simulink model "flatball_6dof"  (R2021b)
settings: Solver=ode1be  StartTime=0.0  StopTime=30  FixedStep=1e-3  MaxStep=0.01  MinStep=0.01  RelTol=1e-3
values from neighbouring files (symbols this model uses):
  amb = evalin( 'base', 'amb')    [flatball_6dof_eqom.m]
  C = evalin( 'base', 'C')    [flatball_6dof_eqom.m]
  disc = evalin( 'base', 'disc')    [flatball_6dof_eqom.m]    (also in flatball_6dof_init.m = struct; flatball_init_disc_params.m = struct)
  X0_z1m_at_rest = [1e-3 1e-3 -1, -1e-6 1e-6 -1e-6, 0 0 1e-6, 0 0 -1e-6]    [flatball_6dof_wrk.m]    (also in hummel_thesis_mdl_validation.m)
undefined symbols (not defined in the file or in its folder): clock, flatball, flatball_6dof_plnt_lib, HandH
libraries: simulink x6, aerolibanim x3, aerolibnav x3, matrix_library x3, mspfiltlib x1, hucker_lib x1
(part 2 of 3)

== system flatball_6dof/flatball-6dof-HandH/calc-F-M/lab/calc-M/q-inf ==
  X : Inport
  Gain : Gain  Gain=0.5
  Product1 : Product  Inputs=3
  Product2 : Product
  S : Constant  Value=disc.A
  Square : Math  Operator=square  SaturateOnIntegerOverflow=on
  X-to-vel : MATLAB Function  TreatAsAtomicUnit=on
  d : Constant  Value=disc.d
  rho : Constant  Value=amb.rho
  vector-norm : MATLAB Function  TreatAsAtomicUnit=on
  q-inf-S : Outport
  q-inf-S-d : Outport  Port=2
  wires:
  d/1 -> Product2/2
  Product2/1 -> q-inf-S-d/1
  X-to-vel/1(vel) -> vector-norm/1(vec)
  Gain/1 -> q-inf-S/1, Product2/1
  Square/1 -> Product1/1
  S/1 -> Product1/2
  vector-norm/1(norm) -> Square/1
  X/1 -> X-to-vel/1(X)
  rho/1 -> Product1/3
  Product1/1 -> Gain/1

== system flatball_6dof/flatball-6dof-HandH/calc-F-M/lab/helpers/Subsystem ==
  Xdot : Inport
  Display : Display
  Gain : Gain  Gain=-1
  Ground2 : Ground
  Ground3 : Ground
  Ta1 : MATLAB Function  TreatAsAtomicUnit=on
  zero-side-slip-angle : MATLAB Function  TreatAsAtomicUnit=on
  Ta23 : Outport
  wires:
  Ground2/1 -> Ta1/2(theta)
  Gain/1 -> Ta1/3(psi)
  Ground3/1 -> Ta1/1(phi)
  Ta1/1(T) -> Ta23/1  "Ta23"
  zero-side-slip-angle/1(beta) -> Display/1, Gain/1  "beta"
  Xdot/1 -> zero-side-slip-angle/1(Xdot)

== system flatball_6dof/flatball-6dof-HandH/calc-F-M/lab/helpers/Subsystem1 ==
  X1_dot : Inport
  TH1_dot : Inport  Port=2
  TH1 : Inport  Port=3
  Display : Display
  Display1 : Display
  MatrixMultiply : Product  Multiplication=Matrix(*)
  MatrixMultiply1 : Product  Multiplication=Matrix(*)
  transformation-matrices : Subsystem
  w_ : MATLAB Function  TreatAsAtomicUnit=on
  X2_dot : Outport
  TH2_dot : Outport  Port=2
  w~ : Outport  Port=3
  wires:
  MatrixMultiply/1 -> Display/1, X2_dot/1
  MatrixMultiply1/1 -> w_/1(THdot), Display1/1, TH2_dot/1
  transformation-matrices/1(Ta12) -> MatrixMultiply/1
  transformation-matrices/2(Tr12) -> MatrixMultiply1/1
  X1_dot/1 -> MatrixMultiply/2
  TH1_dot/1 -> MatrixMultiply1/2
  TH1/1 -> transformation-matrices/1(TH)
  w_/1(M) -> w~/1  "w_"

== system flatball_6dof/flatball-6dof-HandH/calc-F-M/lab/helpers/Subsystem2 ==
  Xdot : Inport
  Display : Display
  Ground : Ground
  Ground1 : Ground
  Ta2 : MATLAB Function  TreatAsAtomicUnit=on
  angle-of-attack : MATLAB Function  TreatAsAtomicUnit=on
  Ta34 : Outport
  wires:
  Ground1/1 -> Ta2/3(psi)
  Ta2/1(T) -> Ta34/1  "Ta34"
  angle-of-attack/1(alpha) -> Display/1, Ta2/2(theta)  "alpha"
  Xdot/1 -> angle-of-attack/1(Xdot)
  Ground/1 -> Ta2/1(phi)

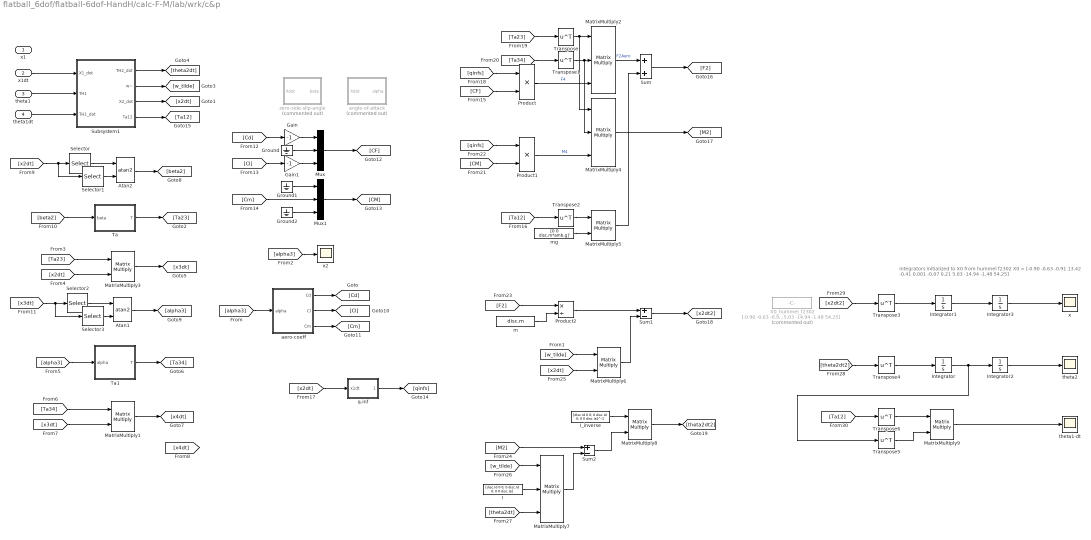
== system flatball_6dof/flatball-6dof-HandH/calc-F-M/lab/wrk/c&p ==
  note: integrators initialized to X0 from hummel f2302
      | X0 = [-0.90 -0.63 -0.91 13.42 -0.41 0.001 -0.07 0.21 5.03 -14.94 -1.48 54.25]
  x1 : Inport
  x1dt : Inport  Port=2
  theta1 : Inport  Port=3
  theta1dt : Inport  Port=4
  Atan1 : Trigonometry  Operator=atan2
  Atan2 : Trigonometry  Operator=atan2
  Gain : Gain  Gain=-1
  Gain1 : Gain  Gain=-1
  Ground : Ground
  Ground1 : Ground
  Ground2 : Ground
  I : Constant  Value=[disc.Id 0 0; 0 disc.Id 0; 0 0 disc.Ia]
  I_inverse : Constant  Value=[disc.Id 0 0; 0 disc.Id 0; 0 0 disc.Ia]^-1
  Integrator : Integrator  InitialCondition=[-14.94 -1.48 54.25]
  Integrator1 : Integrator  InitialCondition=[13.42 -0.41 0.001]
  Integrator2 : Integrator  InitialCondition=[-0.07 0.21 5.03]
  Integrator3 : Integrator  InitialCondition=[-0.90 -0.63 -0.91]
  MatrixMultiply{1,3,5..6,8..9} (6 alike) : Product  Multiplication=Matrix(*)
  MatrixMultiply2 : Product  Inputs=3  Multiplication=Matrix(*)
  MatrixMultiply4 : Product  Inputs=3  Multiplication=Matrix(*)
  MatrixMultiply7 : Product  Inputs=3  Multiplication=Matrix(*)
  Mux : Mux  Inputs=3
  Mux1 : Mux  Inputs=3
  Product : Product
  Product1 : Product
  Product2 : Product  Inputs=*/
  Selector : Selector  InputPortWidth=3  IndexOptions=Index vector (dialog)  Indices=[2]  OutputSizes=1
  Selector1 : Selector  InputPortWidth=3  IndexOptions=Index vector (dialog)  Indices=[1]  OutputSizes=1
  Selector2 : Selector  InputPortWidth=3  IndexOptions=Index vector (dialog)  Indices=[3]  OutputSizes=1
  Selector3 : Selector  InputPortWidth=3  IndexOptions=Index vector (dialog)  Indices=[1]  OutputSizes=1
  Subsystem1 : Subsystem
  Sum : Sum
  Sum1 : Sum  Inputs=+-
  Sum2 : Sum  Inputs=+-
  Ta : MATLAB Function  TreatAsAtomicUnit=on
  Ta1 : MATLAB Function  TreatAsAtomicUnit=on
  Transpose{,1..6} (7 alike) : Math  Operator=transpose  SaturateOnIntegerOverflow=on
  X0_hummel_f2302 : Constant  Commented=on  Value=[-0.90 -0.63 -0.91 13.42 -0.41 0.001 -0.07 0.21 5.03 -14.94 -1.48 54.25]
  aero-coeff : Subsystem
  angle-of-attack : MATLAB Function  Commented=on  TreatAsAtomicUnit=on
  m : Constant  Value=disc.m
  mg : Constant  Value=[0 0 disc.m*amb.g]'
  q-inf : Subsystem
  theta1-dt : Scope
  theta2 : Scope
  x : Scope
  x2 : Scope
  zero-side-slip-angle : MATLAB Function  Commented=on  TreatAsAtomicUnit=on
  wires:
  x1dt/1 -> Subsystem1/1(X1_dot)
  theta1dt/1 -> Subsystem1/3(TH1_dot)
  theta1/1 -> Subsystem1/2(TH1)
  Ta/1(T) -> [Ta23]
  Subsystem1/2(w~) -> [w_tilde]
  Subsystem1/1(TH2_dot) -> [theta2dt]
  [beta2] -> Ta/1(beta)
  MatrixMultiply3/1 -> [x3dt]
  [alpha3] -> Ta1/1(alpha)
  Ta1/1(T) -> [Ta34]
  MatrixMultiply1/1 -> [x4dt]
  [x2dt] -> Selector1/1, Selector/1
  Atan2/1 -> [beta2]
  Atan1/1 -> [alpha3]
  aero-coeff/1(Cd) -> [Cd]
  aero-coeff/3(Cm) -> [Cm]
  aero-coeff/2(Cl) -> [Cl]
  [alpha3] -> aero-coeff/1(alpha)
  [Cd] -> Gain/1
  [Cl] -> Gain1/1
  Ground/1 -> Mux/2
  Mux/1 -> [CF]
  Gain/1 -> Mux/1
  Gain1/1 -> Mux/3
  [Cm] -> Mux1/2
  Ground1/1 -> Mux1/1
  Ground2/1 -> Mux1/3
  Mux1/1 -> [CM]
  [x2dt] -> q-inf/1(x1dt)
  q-inf/1(q-inf-S) -> [qinfs]
  [qinfs] -> Product/1
  [CF] -> Product/2
  [Ta34] -> Transpose1/1
  [Ta23] -> Transpose/1
  Transpose/1 -> MatrixMultiply4/1, MatrixMultiply2/1
  Transpose1/1 -> MatrixMultiply4/2, MatrixMultiply2/2
  Product/1 -> MatrixMultiply2/3  "F4"
  [CM] -> Product1/2
  [qinfs] -> Product1/1
  Product1/1 -> MatrixMultiply4/3  "M4"
  [Ta23] -> MatrixMultiply3/1
  [x2dt] -> MatrixMultiply3/2
  [x3dt] -> MatrixMultiply1/2
  [Ta34] -> MatrixMultiply1/1
  Subsystem1/4(Ta12) -> [Ta12]
  [Ta12] -> Transpose2/1
  Transpose2/1 -> MatrixMultiply5/1
  mg/1 -> MatrixMultiply5/2
  MatrixMultiply2/1 -> Sum/1  "F2Aero"
  MatrixMultiply5/1 -> Sum/2
  Sum/1 -> [F2]
  MatrixMultiply4/1 -> [M2]
  [F2] -> Product2/1
  m/1 -> Product2/2
  Product2/1 -> Sum1/1
  [w_tilde] -> MatrixMultiply6/1
  [x2dt] -> MatrixMultiply6/2
  MatrixMultiply6/1 -> Sum1/2
  Sum1/1 -> [x2dt2]
  [M2] -> Sum2/1
  [theta2dt] -> MatrixMultiply7/3
  [w_tilde] -> MatrixMultiply7/1
  I/1 -> MatrixMultiply7/2
  MatrixMultiply7/1 -> Sum2/2
  MatrixMultiply8/1 -> [theta2dt2]
  [theta2dt2] -> Transpose4/1
  [x2dt2] -> Transpose3/1
  Integrator/1 -> Integrator2/1, Transpose5/1
  Integrator1/1 -> Integrator3/1
  Integrator2/1 -> theta2/1
  Integrator3/1 -> x/1
  I_inverse/1 -> MatrixMultiply8/1
  Sum2/1 -> MatrixMultiply8/2
  Subsystem1/3(X2_dot) -> [x2dt]
  Transpose3/1 -> Integrator1/1
  Transpose4/1 -> Integrator/1
  [alpha3] -> x2/1
  Selector/1 -> Atan2/1
  Selector1/1 -> Atan2/2
  Selector3/1 -> Atan1/2
  Selector2/1 -> Atan1/1
  [x3dt] -> Selector3/1, Selector2/1
  Transpose5/1 -> MatrixMultiply9/2
  [Ta12] -> Transpose6/1
  Transpose6/1 -> MatrixMultiply9/1
  MatrixMultiply9/1 -> theta1-dt/1

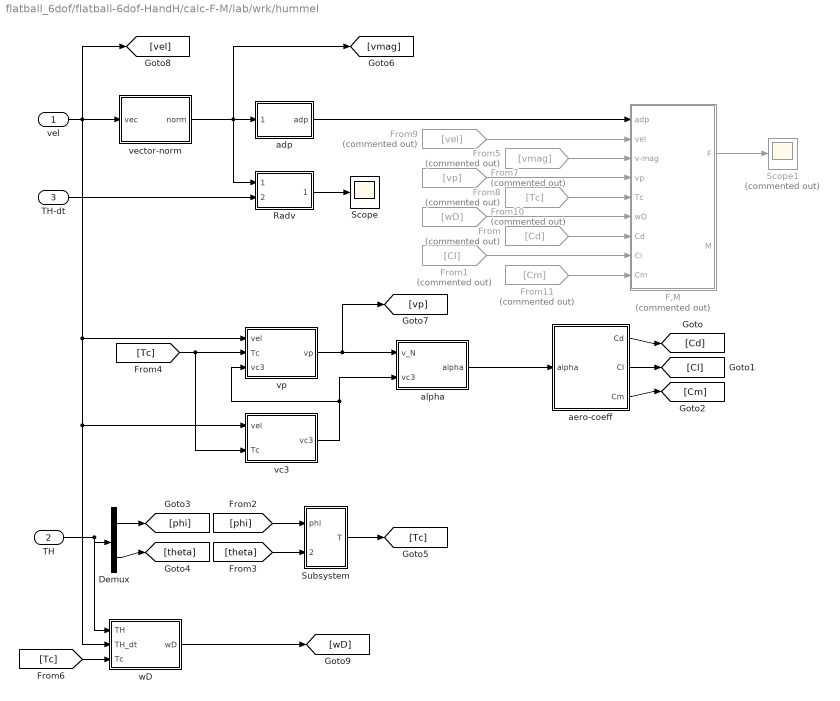
== system flatball_6dof/flatball-6dof-HandH/calc-F-M/lab/wrk/hummel ==
  vel : Inport
  TH : Inport  Port=2
  TH-dt : Inport  Port=3
  Demux : Demux  Outputs=2
  F,M : Subsystem  Commented=on
  From : From  Commented=on  GotoTag=Cd
  From1 : From  Commented=on  GotoTag=Cl
  From10 : From  Commented=on  GotoTag=wD
  From11 : From  Commented=on  GotoTag=Cm
  From5 : From  Commented=on  GotoTag=vmag
  From7 : From  Commented=on  GotoTag=vp
  From8 : From  Commented=on  GotoTag=Tc
  From9 : From  Commented=on  GotoTag=vel
  Radv : Subsystem
  Scope : Scope
  Scope1 : Scope  Commented=on
  Subsystem : Subsystem
  adp : Subsystem
  aero-coeff : Subsystem
  alpha : MATLAB Function  TreatAsAtomicUnit=on
  vc3 : MATLAB Function  TreatAsAtomicUnit=on
  vector-norm : MATLAB Function  TreatAsAtomicUnit=on
  vp : MATLAB Function  TreatAsAtomicUnit=on
  wD : MATLAB Function  TreatAsAtomicUnit=on
  wires:
  aero-coeff/1(Cd) -> [Cd]
  aero-coeff/2(Cl) -> [Cl]
  aero-coeff/3(Cm) -> [Cm]
  adp/1(adp) -> F,M/1(adp)
  vel/1 -> [vel], wD/2(TH_dt), vc3/1(vel), vp/1(vel), vector-norm/1(vec)
  TH/1 -> wD/1(TH), Demux/1
  Demux/2 -> [theta]
  Demux/1 -> [phi]
  [phi] -> Subsystem/1(phi)
  [theta] -> Subsystem/2(theta)
  vector-norm/1(norm) -> Radv/1(v-mag), [vmag], adp/1(v-mag)
  Subsystem/1(T) -> [Tc]
  vp/1(vp) -> [vp], alpha/1(v_N)
  [Tc] -> vc3/2(Tc), vp/2(Tc)
  vc3/1(vc3) -> vp/3(vc3), alpha/2(vc3)
  alpha/1(alpha) -> aero-coeff/1(alpha)
  TH-dt/1 -> Radv/2(TH-dt)
  Radv/1(Radv) -> Scope/1
  [Tc] -> wD/3(Tc)
  wD/1(wD) -> [wD]
  From5/1 -> F,M/3(v-mag)
  From7/1 -> F,M/4(vp)
  From8/1 -> F,M/5(Tc)
  F,M/1(F) -> Scope1/1
  From9/1 -> F,M/2(vel)
  From10/1 -> F,M/6(wD)
  From/1 -> F,M/7(Cd)
  From1/1 -> F,M/8(Cl)
  From11/1 -> F,M/9(Cm)

== system flatball_6dof/flatball-6dof-HandH/scopes/work-in-progress/body-forces-and-moments/mg ==
  Constant1 : Constant  Value=amb.g
  Constant2 : Constant  Value=disc.m
  Ground4 : Ground
  Ground5 : Ground
  Mux2 : Mux  Inputs=3
  Product4 : Product
  mg : Outport
  wires:
  Product4/1 -> mg/1
  Constant1/1 -> Mux2/3
  Ground4/1 -> Mux2/1
  Constant2/1 -> Product4/1
  Mux2/1 -> Product4/2
  Ground5/1 -> Mux2/2

== system flatball_6dof/flatball-6dof-HandH/scopes/work-in-progress/earth-reference/beta2 ==
  X2dot : Inport
  Atan2 : Trigonometry  Operator=atan2
  Selector : Selector  InputPortWidth=3  IndexOptions=Index vector (dialog)  Indices=[2]  OutputSizes=1
  Selector3 : Selector  InputPortWidth=3  IndexOptions=Index vector (dialog)  Indices=[1]  OutputSizes=1
  tag scope: beta2=scoped
  wires:
  Atan2/1 -> [beta2]
  Selector/1 -> Atan2/1  "v2"
  Selector3/1 -> Atan2/2  "u2"
  X2dot/1 -> Selector3/1, Selector/1

== system flatball_6dof/flatball-6dof-HandH/scopes/work-in-progress/earth-reference/v_inf ==
  X2dot : Inport
  Demux : Demux  Outputs=3
  Sqrt : Sqrt  SaturateOnIntegerOverflow=on
  Square : Math  Operator=square  SaturateOnIntegerOverflow=on
  Square1 : Math  Operator=square  SaturateOnIntegerOverflow=on
  Square2 : Math  Operator=square  SaturateOnIntegerOverflow=on
  Sum : Sum  Inputs=3
  tag scope: v_inf=scoped
  wires:
  Square1/1 -> Sum/2
  Square2/1 -> Sum/3
  Sum/1 -> Sqrt/1
  Demux/1 -> Square/1
  Square/1 -> Sum/1
  Demux/3 -> Square2/1
  X2dot/1 -> Demux/1
  Demux/2 -> Square1/1
  Sqrt/1 -> [v_inf]

== system flatball_6dof/flatball-6dof-HandH/scopes/work-in-progress/earth-reference/w_tilde ==
  X2dot : Inport
  MATLAB Function : MATLAB Function  TreatAsAtomicUnit=on
  tag scope: w_tilde=scoped
  wires:
  MATLAB Function/1(w) -> [w_tilde]
  X2dot/1 -> MATLAB Function/1(X2dot)

== system flatball_6dof/flatball-6dof-HandH/scopes/work-in-progress/eml-6dof/lab ==
  X1 : Inport
  TH1 : Inport  Port=2
  X1-dot : Inport  Port=3
  TH1-dot : Inport  Port=4
  X2-dot : Inport  Port=5
  TH2-dot : Inport  Port=6
  X3-dot : Inport  Port=7
  TH3-dot : Inport  Port=8
  alpha3 : Inport  Port=9
  beta2 : Inport  Port=10
  Compare To Constant : simulink/Logic and Bit Operations/Compare To Constant  relop=>=  const=0.0  OutDataTypeStr=boolean
  Gain : Gain  Gain=C.RAD2DEG
  Gain1 : Gain  Gain=C.RAD2DEG
  Scope{,1..9} (10 alike) : Scope
  Selector : Selector  InputPortWidth=3  IndexOptions=Index vector (dialog)  Indices=[3]  OutputSizes=1
  Selector1 : Selector  InputPortWidth=3  IndexOptions=Index vector (dialog)  Indices=[1 2]  OutputSizes=1
  Stop Simulation : Stop
  wires:
  Selector1/1 -> Scope1/1
  Gain1/1 -> Scope9/1
  Gain/1 -> Scope8/1
  Selector/1 -> Compare To Constant/1
  Compare To Constant/1 -> Stop Simulation/1
  TH3-dot/1 -> Scope7/1
  TH1-dot/1 -> Scope3/1
  TH2-dot/1 -> Scope5/1
  X2-dot/1 -> Scope4/1
  TH1/1 -> Selector1/1
  X1/1 -> Scope/1, Selector/1
  beta2/1 -> Gain1/1
  X3-dot/1 -> Scope6/1
  X1-dot/1 -> Scope2/1
  alpha3/1 -> Gain/1

== system flatball_6dof/flatball-6dof-HandH/calc-F-M/lab/calc-F/aero-coeff/Subsystem ==
  alpha : Inport
  Cd0 : Constant  Value=disc.CD0
  Cda : Constant  Value=disc.CDa
  Product : Product
  Square : Math  Operator=square  SaturateOnIntegerOverflow=on
  Sum : Sum
  Sum1 : Sum
  alpha0 : Constant  Value=disc.alpha0
  Cd : Outport
  wires:
  Sum1/1 -> Cd/1
  Square/1 -> Product/2
  Product/1 -> Sum1/2
  Cda/1 -> Product/1
  Cd0/1 -> Sum1/1
  Sum/1 -> Square/1
  alpha0/1 -> Sum/2
  alpha/1 -> Sum/1

== system flatball_6dof/flatball-6dof-HandH/calc-F-M/lab/calc-F/aero-coeff/Subsystem1 ==
  alpha : Inport
  CL0 : Constant  Value=disc.CL0
  CLa : Constant  Value=disc.CLa
  Product : Product
  Sum1 : Sum
  Cl : Outport
  wires:
  alpha/1 -> Product/2
  CL0/1 -> Sum1/1
  CLa/1 -> Product/1
  Product/1 -> Sum1/2
  Sum1/1 -> Cl/1

== system flatball_6dof/flatball-6dof-HandH/calc-F-M/lab/calc-M/aero-coeff/Subsystem2 ==
  alpha : Inport
  CM0 : Constant  Value=disc.CM0
  CMa : Constant  Value=disc.CMa
  Product : Product
  Sum1 : Sum
  Cm : Outport
  wires:
  Sum1/1 -> Cm/1
  Product/1 -> Sum1/2
  CMa/1 -> Product/1
  CM0/1 -> Sum1/1
  alpha/1 -> Product/2

== system flatball_6dof/flatball-6dof-HandH/calc-F-M/lab/helpers/Subsystem1/transformation-matrices ==
  TH : Inport
  Ta : MATLAB Function  TreatAsAtomicUnit=on
  Tr : MATLAB Function  TreatAsAtomicUnit=on
  Ta12 : Outport
  Tr12 : Outport  Port=2
  wires:
  TH/1 -> Ta/1(TH), Tr/1(TH)
  Ta/1(M) -> Ta12/1  "Ta12"
  Tr/1(M) -> Tr12/1  "Tr12"

== system flatball_6dof/flatball-6dof-HandH/calc-F-M/lab/wrk/c&p/Subsystem1 ==
  X1_dot : Inport
  TH1 : Inport  Port=2
  TH1_dot : Inport  Port=3
  MatrixMultiply : Product  Multiplication=Matrix(*)
  MatrixMultiply1 : Product  Multiplication=Matrix(*)
  Transpose : Math  Operator=transpose  SaturateOnIntegerOverflow=on
  Transpose1 : Math  Operator=transpose  SaturateOnIntegerOverflow=on
  transformation-matrices : Subsystem
  w_ : MATLAB Function  TreatAsAtomicUnit=on
  TH2_dot : Outport
  w~ : Outport  Port=2
  X2_dot : Outport  Port=3
  Ta12 : Outport  Port=4
  wires:
  MatrixMultiply/1 -> X2_dot/1
  MatrixMultiply1/1 -> w_/1(THdot), TH2_dot/1
  transformation-matrices/1(Ta12) -> Transpose/1, Ta12/1
  transformation-matrices/2(Tr12) -> Transpose1/1
  X1_dot/1 -> MatrixMultiply/2
  TH1_dot/1 -> MatrixMultiply1/2
  TH1/1 -> transformation-matrices/1(TH)
  w_/1(M) -> w~/1  "w_"
  Transpose/1 -> MatrixMultiply/1  "Ta21"
  Transpose1/1 -> MatrixMultiply1/1  "Ta21"

== system flatball_6dof/flatball-6dof-HandH/calc-F-M/lab/wrk/c&p/aero-coeff ==
  alpha : Inport
  Subsystem : Subsystem
  Subsystem1 : Subsystem
  Subsystem2 : Subsystem
  Cd : Outport
  Cl : Outport  Port=2
  Cm : Outport  Port=3
  wires:
  alpha/1 -> Subsystem2/1(alpha), Subsystem1/1(alpha), Subsystem/1(alpha)
  Subsystem2/1(Cm) -> Cm/1
  Subsystem1/1(Cl) -> Cl/1
  Subsystem/1(Cd) -> Cd/1

== system flatball_6dof/flatball-6dof-HandH/calc-F-M/lab/wrk/c&p/q-inf ==
  x1dt : Inport
  Gain : Gain  Gain=0.5
  Product1 : Product  Inputs=3
  S : Constant  Value=disc.A
  Square : Math  Operator=square  SaturateOnIntegerOverflow=on
  rho : Constant  Value=amb.rho
  vector-norm : MATLAB Function  TreatAsAtomicUnit=on
  q-inf-S : Outport
  wires:
  Product1/1 -> Gain/1
  rho/1 -> Product1/3
  x1dt/1 -> vector-norm/1(vec)
  vector-norm/1(norm) -> Square/1
  S/1 -> Product1/2
  Square/1 -> Product1/1
  Gain/1 -> q-inf-S/1

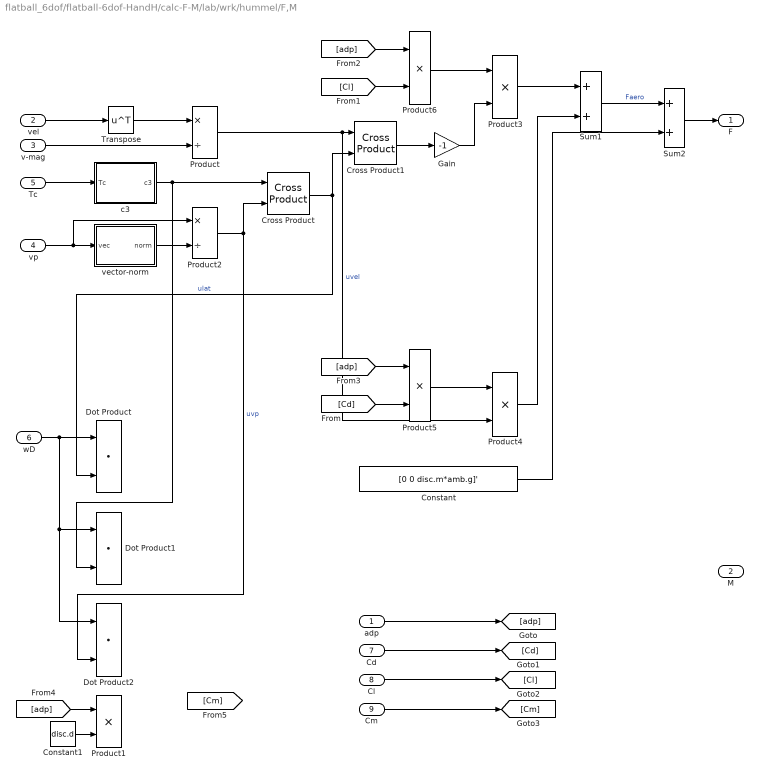
== system flatball_6dof/flatball-6dof-HandH/calc-F-M/lab/wrk/hummel/F,M ==
  adp : Inport
  vel : Inport  Port=2
  v-mag : Inport  Port=3
  vp : Inport  Port=4
  Tc : Inport  Port=5
  wD : Inport  Port=6
  Cd : Inport  Port=7
  Cl : Inport  Port=8
  Cm : Inport  Port=9
  Constant : Constant  Value=[0 0 disc.m*amb.g]'
  Constant1 : Constant  Value=disc.d
  Cross Product : matrix_library/Cross Product
      settings: SourceProductBaseCode=SL
  Cross Product1 : matrix_library/Cross Product
      settings: SourceProductBaseCode=SL
  Dot Product : DotProduct  InputSameDT=on  OutDataTypeStr=Inherit: Inherit via internal rule
  Dot Product1 : DotProduct  InputSameDT=on  OutDataTypeStr=Inherit: Inherit via internal rule
  Dot Product2 : DotProduct  InputSameDT=on  OutDataTypeStr=Inherit: Inherit via internal rule
  Gain : Gain  Gain=-1
  Product : Product  Inputs=*/
  Product1 : Product  Inputs=**
  Product2 : Product  Inputs=*/
  Product{3..6} (4 alike) : Product
  Sum1 : Sum
  Sum2 : Sum
  Transpose : Math  Operator=transpose  SaturateOnIntegerOverflow=on
  c3 : MATLAB Function  TreatAsAtomicUnit=on
  vector-norm : MATLAB Function  TreatAsAtomicUnit=on
  F : Outport
  M : Outport  Port=2
  wires:
  vel/1 -> Transpose/1
  v-mag/1 -> Product/2
  vp/1 -> Product2/1, vector-norm/1(vec)
  vector-norm/1(norm) -> Product2/2
  Product2/1 -> Dot Product2/2, Cross Product/2  "uvp"
  Tc/1 -> c3/1(Tc)
  c3/1(c3) -> Dot Product1/2, Cross Product/1
  Cross Product/1 -> Cross Product1/2, Dot Product/2  "ulat"
  Product/1 -> Cross Product1/1, Product4/2  "uvel"
  Cross Product1/1 -> Gain/1
  Gain/1 -> Product3/2
  Product3/1 -> Sum1/1
  Product4/1 -> Sum1/2
  Sum1/1 -> Sum2/1  "Faero"
  Transpose/1 -> Product/1
  Sum2/1 -> F/1
  Constant/1 -> Sum2/2
  adp/1 -> [adp]
  Constant1/1 -> Product1/2
  wD/1 -> Dot Product2/1, Dot Product1/1, Dot Product/1
  Product5/1 -> Product4/1
  [Cl] -> Product6/2
  [Cd] -> Product5/2
  Product6/1 -> Product3/1
  [adp] -> Product6/1
  [adp] -> Product5/1
  Cd/1 -> [Cd]
  Cl/1 -> [Cl]
  Cm/1 -> [Cm]
  [adp] -> Product1/1

== system flatball_6dof/flatball-6dof-HandH/calc-F-M/lab/wrk/hummel/Radv ==
  v-mag : Inport
  TH-dt : Inport  Port=2
  Gain : Gain  Gain=0.5
  Product1 : Product  Inputs=**/
  Selector : Selector  InputPortWidth=3  IndexOptions=Index vector (dialog)  Indices=[3]  OutputSizes=1
  "[0.5 .. inf]" : Saturate  UpperLimit=inf  LowerLimit=0.50
  d : Constant  Value=disc.d
  Radv : Outport
  wires:
  Product1/1 -> Radv/1
  d/1 -> Gain/1
  TH-dt/1 -> Selector/1
  Selector/1 -> Product1/1
  Gain/1 -> Product1/2
  v-mag/1 -> "[0.5 .. inf]"/1
  "[0.5 .. inf]"/1 -> Product1/3

== system flatball_6dof/flatball-6dof-HandH/calc-F-M/lab/wrk/hummel/Subsystem ==
  phi : Inport
  theta : Inport  Port=2
  Tc : MATLAB Function  TreatAsAtomicUnit=on
  T : Outport
  wires:
  theta/1 -> Tc/2(theta)
  phi/1 -> Tc/1(phi)
  Tc/1(Tc) -> T/1

== system flatball_6dof/flatball-6dof-HandH/calc-F-M/lab/wrk/hummel/adp ==
  v-mag : Inport
  A : Constant  Value=disc.A
  Gain : Gain  Gain=0.5
  Product : Product
  Product1 : Product  Inputs=3
  rho : Constant  Value=amb.rho
  adp : Outport
  wires:
  Product1/1 -> adp/1
  rho/1 -> Product/1
  A/1 -> Product/2
  Product/1 -> Gain/1
  v-mag/1 -> Product1/2, Product1/1
  Gain/1 -> Product1/3

== system flatball_6dof/flatball-6dof-HandH/calc-F-M/lab/wrk/hummel/aero-coeff ==
  alpha : Inport
  Subsystem : Subsystem
  Subsystem1 : Subsystem
  Subsystem2 : Subsystem
  Cd : Outport
  Cl : Outport  Port=2
  Cm : Outport  Port=3
  wires:
  alpha/1 -> Subsystem2/1(alpha), Subsystem1/1(alpha), Subsystem/1(alpha)
  Subsystem2/1(Cm) -> Cm/1
  Subsystem1/1(Cl) -> Cl/1
  Subsystem/1(Cd) -> Cd/1

== system flatball_6dof/flatball-6dof-HandH/calc-F-M/lab/wrk/c&p/Subsystem1/transformation-matrices ==
  TH : Inport
  Ta : MATLAB Function  TreatAsAtomicUnit=on
  Tr : MATLAB Function  TreatAsAtomicUnit=on
  Ta12 : Outport
  Tr12 : Outport  Port=2
  wires:
  TH/1 -> Ta/1(TH), Tr/1(TH)
  Ta/1(Ta12) -> Ta12/1
  Tr/1(Tr12) -> Tr12/1

== system flatball_6dof/flatball-6dof-HandH/calc-F-M/lab/wrk/c&p/aero-coeff/Subsystem ==
  alpha : Inport
  Cd0 : Constant  Value=disc.CD0
  Cda : Constant  Value=disc.CDa
  Product : Product
  Square : Math  Operator=square  SaturateOnIntegerOverflow=on
  Sum : Sum
  Sum1 : Sum
  alpha0 : Constant  Value=disc.alpha0
  Cd : Outport
  wires:
  Sum1/1 -> Cd/1
  Square/1 -> Product/2
  Product/1 -> Sum1/2
  Cda/1 -> Product/1
  Cd0/1 -> Sum1/1
  Sum/1 -> Square/1
  alpha0/1 -> Sum/2
  alpha/1 -> Sum/1

== system flatball_6dof/flatball-6dof-HandH/calc-F-M/lab/wrk/c&p/aero-coeff/Subsystem1 ==
  alpha : Inport
  CL0 : Constant  Value=disc.CL0
  CLa : Constant  Value=disc.CLa
  Product : Product
  Sum1 : Sum
  Cl : Outport
  wires:
  alpha/1 -> Product/2
  CL0/1 -> Sum1/1
  CLa/1 -> Product/1
  Product/1 -> Sum1/2
  Sum1/1 -> Cl/1

== system flatball_6dof/flatball-6dof-HandH/calc-F-M/lab/wrk/c&p/aero-coeff/Subsystem2 ==
  alpha : Inport
  CM0 : Constant  Value=disc.CM0
  CMa : Constant  Value=disc.CMa
  Product : Product
  Sum1 : Sum
  Cm : Outport
  wires:
  Sum1/1 -> Cm/1
  Product/1 -> Sum1/2
  CMa/1 -> Product/1
  CM0/1 -> Sum1/1
  alpha/1 -> Product/2

== system flatball_6dof/flatball-6dof-HandH/calc-F-M/lab/wrk/hummel/aero-coeff/Subsystem ==
  alpha : Inport
  Cd0 : Constant  Value=disc.CD0
  Cda : Constant  Value=disc.CDa
  Product : Product
  Square : Math  Operator=square  SaturateOnIntegerOverflow=on
  Sum : Sum
  Sum1 : Sum
  alpha0 : Constant  Value=disc.alpha0
  Cd : Outport
  wires:
  Sum1/1 -> Cd/1
  Square/1 -> Product/2
  Product/1 -> Sum1/2
  Cda/1 -> Product/1
  Cd0/1 -> Sum1/1
  Sum/1 -> Square/1
  alpha0/1 -> Sum/2
  alpha/1 -> Sum/1

== system flatball_6dof/flatball-6dof-HandH/calc-F-M/lab/wrk/hummel/aero-coeff/Subsystem1 ==
  alpha : Inport
  CL0 : Constant  Value=disc.CL0
  CLa : Constant  Value=disc.CLa
  Product : Product
  Sum1 : Sum
  Cl : Outport
  wires:
  alpha/1 -> Product/2
  CL0/1 -> Sum1/1
  CLa/1 -> Product/1
  Product/1 -> Sum1/2
  Sum1/1 -> Cl/1

== system flatball_6dof/flatball-6dof-HandH/calc-F-M/lab/wrk/hummel/aero-coeff/Subsystem2 ==
  alpha : Inport
  CM0 : Constant  Value=disc.CM0
  CMa : Constant  Value=disc.CMa
  Product : Product
  Sum1 : Sum
  Cm : Outport
  wires:
  Sum1/1 -> Cm/1
  Product/1 -> Sum1/2
  CMa/1 -> Product/1
  CM0/1 -> Sum1/1
  alpha/1 -> Product/2

== matlab function flatball_6dof/flatball-6dof-HandH/calc-F-M/lab/helpers/Subsystem2/angle-of-attack ==
  data: Xdot input; alpha output
function alpha  = f( Xdot)
% calculate angle of attack

alpha = atan( Xdot(3) / Xdot(1));

== matlab function flatball_6dof/flatball-6dof-HandH/calc-F-M/calc-M/X-to-wD_N_inC ==
  data: TH input; wD_N_inC output; dTHdt input
function wD_N_inC  = f( TH, dTHdt)
%% internal states
theta = TH(2);
p = dTHdt(1); q = dTHdt(2); r = dTHdt(3);

wD_N_inC = [p*cos(theta) q p*sin(theta)+r]';

== matlab function flatball_6dof/flatball-6dof-HandH/calc-F-M/lab/wrk/hummel/vector-norm ==
  data: vec input; norm output
function norm = fcn( vec)

norm = sqrt( vec(1)*vec(1) + vec(2)*vec(2) + vec(3)*vec(3));

== matlab function flatball_6dof/flatball-6dof-HandH/calc-F-M/lab/wrk/hummel/Subsystem/Tc ==
  data: phi input; theta input; Tc output
function Tc = fcn( phi, theta)

sin_theta = sin( theta);
cos_theta = cos( theta);
sin_phi = sin( phi);
cos_phi = cos(phi);

Tc = [
    cos_theta sin_theta*sin_phi -sin_theta*cos_phi;
    0 cos_phi sin_phi;
    sin_theta -cos_theta*sin_phi cos_theta*cos_phi;
    ];

== matlab function flatball_6dof/flatball-6dof-HandH/calc-F-M/lab/wrk/hummel/vp ==
  data: vel input; vp output; Tc input; vc3 input
function vp = fcn( vel, Tc, vc3)

c3 = Tc(:,3);

vp = [ vel - vc3*c3];

== matlab function flatball_6dof/flatball-6dof-HandH/calc-F-M/lab/wrk/hummel/alpha ==
  data: v_N input; vc3 input; alpha output
function alpha = fcn( v_N, vc3)

alpha = atan( vc3 / norm( v_N)); % angle of attack

== matlab function flatball_6dof/flatball-6dof-HandH/calc-F-M/lab/wrk/hummel/vc3 ==
  data: vel input; vc3 output; Tc input
function vc3 = fcn( vel, Tc)

c3 = Tc(:,3);
vc3 = dot( vel, c3);

== matlab function flatball_6dof/flatball-6dof-HandH/calc-F-M/lab/wrk/c&p/Ta ==
  data: beta input; T output
function T  = Ta23( beta)
% transformation matrix
%

cos_beta = cos( beta);
sin_beta = sin( beta);

T = [ ...
    cos_beta -sin_beta 0;
    -sin_beta cos_beta 0;
    0 0 1;
    ];

== matlab function flatball_6dof/flatball-6dof-HandH/calc-F-M/lab/wrk/hummel/F,M/vector-norm ==
  data: vec input; norm output
function norm = fcn( vec)

norm = sqrt( vec(1)*vec(1) + vec(2)*vec(2) + vec(3)*vec(3));

== matlab function flatball_6dof/flatball-6dof-HandH/calc-F-M/lab/wrk/hummel/F,M/c3 ==
  data: Tc input; c3 output
function c3 = fcn( Tc)

c3 = Tc(:,3);

== matlab function flatball_6dof/flatball-6dof-HandH/calc-F-M/lab/wrk/hummel/wD ==
  data: TH input; TH_dt input; wD output; Tc input
function wD = fcn( TH, TH_dt, Tc)

cos_theta = cos( TH(2));
sin_theta = sin( TH(2));

phidot = TH_dt(1);
thetadot = TH_dt(2);
gammadot = TH_dt(3);

wD_N_inC = [phidot*cos_theta thetadot phidot*sin_theta+gammadot];
wD = Tc' * wD_N_inC';

== matlab function flatball_6dof/flatball-6dof-HandH/calc-F-M/lab/wrk/c&p/q-inf/vector-norm ==
  data: vec input; norm output
function norm = fcn( vec)

norm = sqrt( vec(1)*vec(1) + vec(2)*vec(2) + vec(3)*vec(3));

== matlab function flatball_6dof/flatball-6dof-HandH/calc-F-M/lab/wrk/c&p/Subsystem1/transformation-matrices/Ta ==
  data: TH input; Ta12 output
function Ta12  = Ta( TH)
% transformation matrix
%
phi = TH(1); theta = TH(2); psi = TH(3);

cos_phi = cos( phi);
cos_theta = cos( theta);
cos_psi = cos( psi);

sin_phi = sin( phi);
sin_theta = sin( theta);
sin_psi = sin( psi);

Ta12 = [ ...
    cos_theta*cos_psi sin_phi*sin_theta*cos_phi-cos_phi*sin_psi cos_phi*sin_theta*cos_psi+sin_phi*sin_psi;
    cos_theta*sin_psi sin_phi*sin_theta*sin_psi+cos_phi*cos_psi cos_phi*sin_theta*sin_psi-sin_phi*cos_psi;
    -sin_theta sin_phi*cos_theta cos_phi*cos_theta
    ];

% cos_neg_phi = cos( -phi);
% cos_neg_theta = cos( -theta);
% cos_neg_psi = cos( -psi);
% 
% sin_neg_phi = sin( -phi);
% sin_neg_theta = sin( -theta);
% sin_neg_psi = sin( -psi);
% 
% Ta12 = [ ...
%     cos_neg_theta*cos_neg_psi sin_neg_phi*sin_neg_theta*cos_neg_phi-cos_neg_phi*sin_neg_psi cos_neg_phi*sin_neg_theta*cos_neg_psi+sin_neg_phi*sin_neg_psi;
%     cos_neg_theta*sin_neg_psi sin_neg_phi*sin_neg_theta*sin_neg_psi+cos_neg_phi*cos_neg_psi cos_neg_phi*sin_neg_theta*sin_neg_psi-sin_neg_phi*cos_neg_psi;
%     -sin_neg_theta sin_neg_phi*cos_neg_theta cos_neg_phi*cos_neg_theta
%     ];

== matlab function flatball_6dof/flatball-6dof-HandH/calc-F-M/lab/wrk/c&p/Subsystem1/transformation-matrices/Tr ==
  data: TH input; Tr12 output
function Tr12  = Tr( TH)
% transformation matrix
%
phi = TH(1); theta = TH(2); psi = TH(3);

cos_phi = cos( phi);
cos_theta = cos( theta);
cos_psi = cos( psi);

sin_phi = sin( phi);
sin_theta = sin( theta);
sin_psi = sin( psi);

Tr12 = [
    1 0 -sin_theta;
    0 cos_phi cos_theta*sin_psi;
    0 -sin_phi cos_theta*cos_psi;
    ];

== matlab function flatball_6dof/flatball-6dof-HandH/calc-F-M/lab/wrk/c&p/Subsystem1/w_ ==
  data: THdot input; M output
function M  = w_( THdot)
% transformation matrix
%
p = THdot(1); q = THdot(2); r = THdot(3);

M = [ ...
    0 -r q;
    r 0 -p;
    -q p 0
    ];

== matlab function flatball_6dof/flatball-6dof-HandH/calc-F-M/lab/wrk/c&p/Ta1 ==
  data: alpha input; T output
function T  = Ta34( alpha)
% transformation matrix
%

cos_alpha = cos( alpha);
sin_alpha = sin( alpha);

T= [ ...
    cos_alpha 0 -sin_alpha;
    0 1 0;
    sin_alpha 0 cos_alpha;
    ];

== matlab function flatball_6dof/flatball-6dof-HandH/calc-F-M/lab/wrk/c&p/angle-of-attack ==
  data: Xdot input; alpha output
function alpha  = f( Xdot)
% calculate angle of attack

alpha = atan2( Xdot(3) / Xdot(1));

== matlab function flatball_6dof/flatball-6dof-HandH/calc-F-M/lab/wrk/c&p/zero-side-slip-angle ==
  data: Xdot input; beta output
function beta  = f( Xdot)
% calculate side-slip angle

y = Xdot(2);
x = Xdot(1);

beta = atan2( y / x);

== matlab function flatball_6dof/flatball-6dof-HandH/calc-F-M/lab/wrk/flatball_6dof_v1p1 ==
  data: X input; Xdot output; lift output; drag output; alpha output; AdvR output; E_trans output; E_rot output
function [Xdot, lift, drag, alpha, AdvR, E_trans, E_rot]  = flatball_6dof_eom( X)
% flatball equations of motion - NED (north-east-down) configuration
%

%% internal states
x = X(1); y = X(2); z = X(3);
xdot = X(4); ydot = X(5); zdot = X(6);

phi = X(7); theta = X(8); gamma = X(9);
phidot = X(10); thetadot = X(11); gammadot = X(12);

Xdot = zeros(1,12);

%% define ambient parameters
amb.g = 9.81; % m/s^2
amb.rho = 1.23; % Kg/m^3

%% define non-aerodynamic parameters
disc = struct;
disc.m = 0.175; % Kg
disc.A = 0.057; % m^2
disc.d = 2*sqrt(0.057/pi); % 2*sqrt(disc.A/pi); % diameter
disc.Ia = 0.002352; % moment of inertia about the spinning axis
disc.Id = 0.001219; % moment of inertia about the planar axis'

%% crowther and potts - per hummel and hubbard
% disc.CL0 = 0.13;
% disc.CLa = 3.09;
% disc.CD0 = 0.085;
% disc.CDa = 3.30;
% disc.CM0 = -0.01;
% disc.CMa = 0.057;
% 
% disc.CMq = 0.0008; % NOTE: not used
% disc.CLr = 0.0004;
% disc.CLp = -0.013;
% disc.CNr = -2.8e-5;
% 
% disc.alpha0 = -0.052; % rad

%% hummel and hubbard 2014
disc.CL0 = 0.188;
disc.CLa = 2.37;

disc.CD0 = 0.15;
disc.CDa = 1.24;

disc.CM0 = -0.06;
disc.CMa = 0.38;

disc.CMq = 0.0008; % NOTE: not used
disc.CLr = 0.0004;

disc.CNr = -2.8e-5;

disc.CLp = -0.013;

% disc.CRr = 1.4e-2; % NOTE: missing from 2014, borrowed from 2003 thesis
% disc.CRr = 3e-3; % NOTE: missing from 2014, borrowed from P&C
disc.CRr = 0.00171; % appendix of hummel thesis
disc.CRp =-5.5e-3; % NOTE: missing from 2014, borrowed from P&C

% not sure where these are from...
% disc.CMq= -1.44E-02;
% disc.CRp =-1.25E-02;
% disc.CNr = -3.41E-05; % long flight f2302

disc.alpha0 = -0.052; % rad

%% helper variables
sin_theta = sin( theta);
cos_theta = cos( theta);
sin_phi = sin( phi);
cos_phi = cos(phi);

% c = T_c_N * N --> transformation matrix T_c_N in N reference frame
T_c_N = [cos_theta sin_theta*sin_phi -sin_theta*cos_phi;
    0 cos_phi sin_phi;
    sin_theta -cos_theta*sin_phi cos_theta*cos_phi];
% c1 = T_c_N(1,:);
% c2 = T_c_N(2,:);
c3 = T_c_N(3,:);

%% aerodynamic forces and moments in N reference frame
vel = [xdot ydot zdot];
vmag = norm( vel);
vc3 = dot( vel, c3);
v_N = [ vel - vc3*c3];
Adp = 0.5 * disc.A * amb.rho * vmag*vmag;
uvel = vel / vmag;
uv_N = v_N / norm( v_N);
u_lat = cross( c3, uv_N);

wD_N_inC = [phidot*cos_theta thetadot phidot*sin_theta+gammadot];
wD_N_inN = T_c_N' * wD_N_inC';

w_v_N = dot( wD_N_inN, uv_N);
w_lat = dot( wD_N_inN, u_lat);
w_spin = dot( wD_N_inN, c3);

alpha = atan( vc3 / norm( v_N)); % angle of attack
AdvR = disc.d * w_spin / 2 / vmag; % advance ratio
E_trans = 0.5 * disc.m * vmag*vmag; % translational energy
E_rot = 0.5 * disc.Ia * gammadot*gammadot; % rotational energy

%% hacks
k_spin_down_decay = 0.25;
% k_CL_gain = 1.0; %2.5;
% k_CD_gain = 1.0; %1.5;
% k_M_gain = 1.0;

%% coefficients - f(alpha)
dalpha = alpha - disc.alpha0;
CL = disc.CL0 + disc.CLa * alpha;
CD = disc.CD0 + disc.CDa * dalpha*dalpha;
CM = disc.CM0 + disc.CMa * alpha;
Mv_N = Adp * disc.d * (sqrt(disc.d/amb.g)*disc.CRr*w_spin + disc.CRp*w_v_N) * uv_N;

%% coefficients - lookup based
% 
% CL = interp1( disc.CL_data(:,1), disc.CL_data(:,2).*k_CL_gain, alpha, 'spline');
% CD = interp1( disc.CD_data(:,1), disc.CD_data(:,2).*k_CD_gain, alpha, 'spline');
% CM = interp1( disc.CM_data(:,1), disc.CM_data(:,2).*k_M_gain, alpha, 'spline');
% % CRr = interp2( disc.CRr_rad, disc.CRr_AdvR, disc.CRr_data, alpha, AdvR,'spline');
% Mv_N = Adp * disc.d * ( disc.CRr* + disc.CRp*w_v_N) * uv_N;

%%
lift = CL * Adp;
drag = CD * Adp;
ulift = -cross( uvel, u_lat);
udrag = -uvel;
Faero = lift*ulift + drag*udrag;
Fg_N = [0 0 disc.m*amb.g]';

F = Faero' + Fg_N;

Mlat = Adp * disc.d * (CM + disc.CMq * w_lat) * u_lat;
Mspin = [0 0 disc.CNr*w_spin];
M = T_c_N * Mv_N' + T_c_N*Mlat' + Mspin';

%%
xdotdot = F(1) / disc.m;
ydotdot = F(2) / disc.m;
zdotdot = F(3) / disc.m;

phidotdot = (M(1) + disc.Id*thetadot*phidot*sin_theta - disc.Ia*thetadot*(phidot*sin_theta+gammadot) + disc.Id*thetadot*phidot*sin_theta)/disc.Id/cos_theta; 
thetadotdot = (M(2) + disc.Ia*phidot*cos_theta*(phidot*sin_theta +gammadot) - disc.Id*phidot*phidot*cos_theta*sin_theta)/disc.Id;
gammadotdot = (M(3) - disc.Ia*(k_spin_down_decay*gammadot*sin_theta + thetadot*phidot*cos_theta))/disc.Ia;

% bug in hummels report?
% gammadotdot = (M(3) - disc.Ia*(phidotdot*sin_theta + thetadot*phidot*cos_theta))/disc.Ia;
% bug in hummels report?
% w/phidotdot term, there is no decay in gammadot
% w/out gammadot term - there is no decay in gammadot
% NOTE: w/it, the decay is too agressive
% FIXME: investigate why this term is necessary for more appropriate
% spindown (based on my data)

%%
Xdot(1) = xdot;
Xdot(2) = ydot;
Xdot(3) = zdot;

Xdot(4) = xdotdot;
Xdot(5) = ydotdot;
Xdot(6) = zdotdot;

Xdot(7) = phidot;
Xdot(8) = thetadot;
Xdot(9) = gammadot;

Xdot(10) = phidotdot;
Xdot(11) = thetadotdot;
Xdot(12) = gammadotdot;

== matlab function flatball_6dof/flatball-6dof-HandH/calc-F-M/lab/rotations/X-to-T_c_N ==
  data: X input; T_c_N output
function T_c_N  = f( X)
%% internal states
phi = X(7); theta = X(8);

%% helper variables
sin_theta = sin( theta);
cos_theta = cos( theta);
sin_phi = sin( phi);
cos_phi = cos(phi);

T_c_N = [
    cos_theta sin_theta*sin_phi -sin_theta*cos_phi;
    0 cos_phi sin_phi;
    sin_theta -cos_theta*sin_phi cos_theta*cos_phi
    ];

== matlab function flatball_6dof/flatball-6dof-HandH/calc-F-M/lab/alpha- ==
  data: X input; alpha output; T_c_N input
function alpha  = f( X, T_c_N)
%% internal states
xdot = X(4); ydot = X(5); zdot = X(6);

%% helper variables
T_c_Npsi = T_c_N(3,:);

vel = [xdot ydot zdot];
vc3 = dot( vel, T_c_Npsi);
v_N = [ vel - vc3*T_c_Npsi];

alpha = atan( vc3 / norm( v_N)); % angle of attack

== matlab function flatball_6dof/flatball-6dof-HandH/calc-F-M/lab/rotations/X-to-wD_N_inC ==
  data: X input; wD_N_inC output
function wD_N_inC  = f( X)
%% internal states
theta = X(8);
phidot = X(10); thetadot = X(11); gammadot = X(12);

%% helper variables
sin_theta = sin( theta);
cos_theta = cos( theta);

wD_N_inC = [phidot*cos_theta thetadot phidot*sin_theta+gammadot];

== matlab function flatball_6dof/flatball-6dof-HandH/calc-F-M/lab/calc-F/q-inf/vector-norm ==
  data: vec input; norm output
function norm = fcn( vec)

norm = sqrt( vec(1)*vec(1) + vec(2)*vec(2) + vec(3)*vec(3));

== matlab function flatball_6dof/flatball-6dof-HandH/calc-F-M/lab/calc-F/q-inf/X-to-vel ==
  data: X input; vel output
function vel = fcn( X)
xdot = X(4); ydot = X(5); zdot = X(6);
vel = [xdot ydot zdot];

== matlab function flatball_6dof/flatball-6dof-HandH/calc-F-M/lab/calc-F/X-to-vel ==
  data: X input; vel output
function vel = fcn( X)
xdot = X(4); ydot = X(5); zdot = X(6);
vel = [xdot ydot zdot];

== matlab function flatball_6dof/flatball-6dof-HandH/calc-F-M/lab/calc-M/X-to-vel ==
  data: X input; vel output
function vel = fcn( X)
xdot = X(4); ydot = X(5); zdot = X(6);
vel = [xdot ydot zdot];

== matlab function flatball_6dof/flatball-6dof-HandH/calc-F-M/lab/calc-F/calc-F ==
  data: vel input; F output; T_c_N input; Fg_N input; CLift input; CDrag input; q_inf_times_S input
function F = fcn( vel, T_c_N, Fg_N, CLift, CDrag, q_inf_times_S)
%%
T_c_Npsi = T_c_N(3,:);

vc3 = dot( vel, T_c_Npsi);
v_N = [ vel - vc3*T_c_Npsi];
vmag = norm( vel);
uvel = vel / vmag;
uv_N = v_N / norm( v_N);
u_lat = cross( T_c_Npsi, uv_N);

lift = CLift * q_inf_times_S;
ulift = -cross( uvel, u_lat);

drag = CDrag * q_inf_times_S;
udrag = -uvel;

Faero = lift*ulift + drag*udrag;

F = Faero' + Fg_N;

== matlab function flatball_6dof/flatball-6dof-HandH/calc-F-M/lab/calc-M/calc-M ==
  data: vel input; M output; T_c_N input; wD_N_inN input; CMpitch input; q_inf_times_Sd input
function M = fcn( vel, T_c_N, wD_N_inN, CMpitch, q_inf_times_Sd)
%% define ambient parameters
amb.g = 9.81; % m/s^2
amb.rho = 1.23; % Kg/m^3

%% define non-aerodynamic parameters
disc = struct;
disc.m = 0.175; % Kg
disc.A = 0.057; % m^2
disc.d = 2*sqrt(0.057/pi); % 2*sqrt(disc.A/pi); % diameter
disc.Ia = 0.002352; % moment of inertia about the spinning axis
disc.Id = 0.001219; % moment of inertia about the planar axis'

%% crowther and potts - per hummel and hubbard
disc.CMq= -1.44e-2;
disc.CNr = -7.1e-6; % short flights
% disc.CNr = -3.41e-5; % long flight f2302
disc.CRr = 3e-3; % NOTE: missing from 2014, borrowed from P&C
disc.CRp =-5.5e-3; % NOTE: missing from 2014, borrowed from P&C
% disc.CLr = 0.0004;
% disc.CLp = -0.013;
% 

%% helper variables
T_c_Npsi = T_c_N(3,:);

%% aerodynamic forces and moments in N reference frame
vc3 = dot( vel, T_c_Npsi);
v_N = [ vel - vc3*T_c_Npsi];

uv_N = v_N / norm( v_N);
u_lat = cross( T_c_Npsi, uv_N);

w_v_N = dot( wD_N_inN, uv_N);
q = dot( wD_N_inN, u_lat);
r = dot( wD_N_inN, T_c_Npsi);
%%
Mv_N = q_inf_times_Sd * (sqrt(disc.d/amb.g)*disc.CRr*r + disc.CRp*w_v_N) * uv_N;
Mpitch = q_inf_times_Sd * (CMpitch + disc.CMq * q) * u_lat;
Mspin = [0 0 disc.CNr*r];
M = T_c_N*Mv_N' + T_c_N*Mpitch' + Mspin';

== matlab function flatball_6dof/flatball-6dof-HandH/calc-F-M/lab/wrk/flatball_6dof_v1p0 ==
  data: X input; Xdot output; lift output; drag output; alpha output; AdvR output; E_trans output; E_rot output
function [Xdot, lift, drag, alpha, AdvR, E_trans, E_rot]  = flatball_6dof_eom( X)
% flatball equations of motion - NED (north-east-down) configuration
%

%% internal states
x = X(1); y = X(2); z = X(3);
xdot = X(4); ydot = X(5); zdot = X(6);

phi = X(7); theta = X(8); gamma = X(9);
phidot = X(10); thetadot = X(11); gammadot = X(12);

Xdot = zeros(1,12);

%% define ambient parameters
amb.g = 9.81; % m/s^2
amb.rho = 1.23; % Kg/m^3

%% define non-aerodynamic parameters
disc = struct;
disc.m = 0.175; % Kg
disc.A = 0.057; % m^2
disc.d = 2*sqrt(0.057/pi); % 2*sqrt(disc.A/pi); % diameter
disc.Ia = 0.002352; % moment of inertia about the spinning axis
disc.Id = 0.001219; % moment of inertia about the planar axis'

disc.alpha0 = -0.052; %-4 * pi/180.0;

%% THE THREE ESTIMATED COEFFICIENTS
disc.CMq= -1.44E-02;
disc.CRp =-1.25E-02;
disc.CNr = -3.41E-05; % long flight f2302

%% THE seven COEFFICIENTS estimated from three flights
disc.CL0= 0.13; %c&p 07
disc.CLa= 3.09; %c&p 07
disc.CD0= 0.085; %c&p 07
disc.CDa= 3.30; %c&p 07
disc.CM0= -0.01; %c&p 07
disc.CMa= 0.057; %c&p 07 
disc.CRr= 0.00171; % for nondimensionalization = sqrt(d/g), magnitude of CRr changes

%% CL =[ rad CL deg]
disc.CL_data=[ -0.1745 -0.2250 -10; ...
-0.05236 0 -3; ...
0 0.150 0; ...
0.08727 0.4500 5; ...
0.17453 0.7250 10; ...
0.26180 0.9750 15; ...
0.34907 1.2000 20; ...
0.43633 1.4500 25; ...
0.52360 1.6750 30];

%% CD =[ rad CD deg]
disc.CD_data=[ -0.1745 0.1500 -10; ...
-0.05236 0.0800 -3; ...
0 0.1000 0; ...
0.08727 0.1500 5; ...
0.1745 0.2600 10; ...
0.26180 0.3900 15; ...
0.3491 0.5700 20; ...
0.4363 0.7500 25; ...
0.5236 0.9200 30];

%% CM =[ rad CM deg]
disc.CM_data=[-0.174532925 -0.0380 -10; ...
-0.087266463 -0.0220 -5; ...
-0.052359878 -0.0140 -3; ...
0 -0.0060 0; ...
0.052359878 -0.0060 3; ...
0.104719755 -0.0020 6; ...
0.157079633 0.0000 9; ...
0.20943951 0.0100 12; ...
0.261799388 0.0220 15; ...
0.34906585 0.0440 20; ...
0.401425728 0.0600 23; ...
0.453785606 0.0840 26; ...
0.523598776 0.1100 30];

%% helper variables
sin_theta = sin( theta);
cos_theta = cos( theta);
sin_phi = sin( phi);
cos_phi = cos(phi);

% c = T_c_N * N --> transformation matrix T_c_N in N reference frame
T_c_N = [cos_theta sin_theta*sin_phi -sin_theta*cos_phi;
    0 cos_phi sin_phi;
    sin_theta -cos_theta*sin_phi cos_theta*cos_phi];
% c1 = T_c_N(1,:);
% c2 = T_c_N(2,:);
c3 = T_c_N(3,:);

%% aerodynamic forces and moments in N reference frame
vel = [xdot ydot zdot];
vmag = norm( vel);
vc3 = dot( vel, c3);
v_N = [ vel - vc3*c3];
Adp = 0.5 * disc.A * amb.rho * vmag*vmag;
uvel = vel / vmag;
uv_N = v_N / norm( v_N);
u_lat = cross( c3, uv_N);

wD_N_inC = [phidot*cos_theta thetadot phidot*sin_theta+gammadot];
wD_N_inN = T_c_N' * wD_N_inC';

w_v_N = dot( wD_N_inN, uv_N);
w_lat = dot( wD_N_inN, u_lat);
w_spin = dot( wD_N_inN, c3);

alpha = atan( vc3 / norm( v_N)); % angle of attack
AdvR = disc.d * w_spin / 2 / vmag; % advance ratio
E_trans = 0.5 * disc.m * vmag*vmag; % translational energy
E_rot = 0.5 * disc.Ia * gammadot*gammadot; % rotational energy

%% hacks
k_spin_down_decay = 0.25;
% k_CL_gain = 1.0; %2.5;
% k_CD_gain = 1.0; %1.5;
% k_M_gain = 1.0;

%% coefficients - f(alpha)
dalpha = alpha - disc.alpha0;
CL = disc.CL0 + disc.CLa * alpha;
CD = disc.CD0 + disc.CDa * dalpha*dalpha;
CM = disc.CM0 + disc.CMa * alpha;
Mv_N = Adp * disc.d * (sqrt(disc.d/amb.g)*disc.CRr*w_spin + disc.CRp*w_v_N) * uv_N;

%% coefficients - lookup based
% 
% CL = interp1( disc.CL_data(:,1), disc.CL_data(:,2).*k_CL_gain, alpha, 'spline');
% CD = interp1( disc.CD_data(:,1), disc.CD_data(:,2).*k_CD_gain, alpha, 'spline');
% CM = interp1( disc.CM_data(:,1), disc.CM_data(:,2).*k_M_gain, alpha, 'spline');
% % CRr = interp2( disc.CRr_rad, disc.CRr_AdvR, disc.CRr_data, alpha, AdvR,'spline');
% Mv_N = Adp * disc.d * ( disc.CRr* + disc.CRp*w_v_N) * uv_N;

%%
lift = CL * Adp;
drag = CD * Adp;
ulift = -cross( uvel, u_lat);
udrag = -uvel;
Faero = lift*ulift + drag*udrag;
Fg_N = [0 0 disc.m*amb.g]';

F = Faero' + Fg_N;

Mlat = Adp * disc.d * (CM + disc.CMq * w_lat) * u_lat;
Mspin = [0 0 disc.CNr*w_spin];
M = T_c_N * Mv_N' + T_c_N*Mlat' + Mspin';

%%
xdotdot = F(1) / disc.m;
ydotdot = F(2) / disc.m;
zdotdot = F(3) / disc.m;

phidotdot = (M(1) + disc.Id*thetadot*phidot*sin_theta - disc.Ia*thetadot*(phidot*sin_theta+gammadot) + disc.Id*thetadot*phidot*sin_theta)/disc.Id/cos_theta; 
thetadotdot = (M(2) + disc.Ia*phidot*cos_theta*(phidot*sin_theta +gammadot) - disc.Id*phidot*phidot*cos_theta*sin_theta)/disc.Id;
gammadotdot = (M(3) - disc.Ia*(k_spin_down_decay*gammadot*sin_theta + thetadot*phidot*cos_theta))/disc.Ia;

% bug in hummels report?
% gammadotdot = (M(3) - disc.Ia*(phidotdot*sin_theta + thetadot*phidot*cos_theta))/disc.Ia;
% bug in hummels report?
% w/phidotdot term, there is no decay in gammadot
% w/out gammadot term - there is no decay in gammadot
% NOTE: w/it, the decay is too agressive
% FIXME: investigate why this term is necessary for more appropriate
% spindown (based on my data)

%%
Xdot(1) = xdot;
Xdot(2) = ydot;
Xdot(3) = zdot;

Xdot(4) = xdotdot;
Xdot(5) = ydotdot;
Xdot(6) = zdotdot;

Xdot(7) = phidot;
Xdot(8) = thetadot;
Xdot(9) = gammadot;

Xdot(10) = phidotdot;
Xdot(11) = thetadotdot;
Xdot(12) = gammadotdot;

== matlab function flatball_6dof/flatball-6dof-HandH/calc-F-M/lab/calc-M/q-inf/X-to-vel ==
  data: X input; vel output
function vel = fcn( X)
xdot = X(4); ydot = X(5); zdot = X(6);
vel = [xdot ydot zdot];

== matlab function flatball_6dof/flatball-6dof-HandH/calc-F-M/lab/calc-M/q-inf/vector-norm ==
  data: vec input; norm output
function norm = fcn( vec)

norm = sqrt( vec(1)*vec(1) + vec(2)*vec(2) + vec(3)*vec(3));

== matlab function flatball_6dof/flatball-6dof-HandH/calc-F-M/lab/internals ==
  data: X input; AdvR output; E_trans output; E_rot output; T_c_N input; wD_N_inN input
function [ AdvR, E_trans, E_rot]  = internals( X, T_c_N, wD_N_inN)
%% internal states
x = X(1); y = X(2); z = X(3);
xdot = X(4); ydot = X(5); zdot = X(6);

phi = X(7); theta = X(8); gamma = X(9);
phidot = X(10); thetadot = X(11); gammadot = X(12);

%% define non-aerodynamic parameters
disc = struct;
disc.m = 0.175; % Kg
disc.A = 0.057; % m^2
disc.d = 2*sqrt(0.057/pi); % 2*sqrt(disc.A/pi); % diameter
disc.Ia = 0.002352; % moment of inertia about the spinning axis
disc.Id = 0.001219; % moment of inertia about the planar axis'

%% helper variables
vel = [xdot ydot zdot];

T_c_Npsi = T_c_N(3,:);

vmag = norm( vel);

r = dot( wD_N_inN, T_c_Npsi);

AdvR = disc.d * r / 2 / vmag; % advance ratio
E_trans = 0.5 * disc.m * vmag*vmag; % translational energy
E_rot = 0.5 * disc.Ia * gammadot*gammadot; % rotational energy

== matlab function flatball_6dof/flatball-6dof-HandH/earth-accelerations/calc-THdot ==
  data: X input; M input; dTHdt2 output
function dTHdt2   = f_rot( X, M)
% flatball equations of motion - NED (north-east-down) configuration
%

%% internal states
phi = X(4); theta = X(5); gamma = X(6);
p = X(10); q = X(11); r = X(12);

dTHdt2 = zeros(3,1);

%% define non-aerodynamic parameters
disc = struct;
disc.Ia = 0.002352; % moment of inertia about the spinning axis
disc.Id = 0.001219; % moment of inertia about the planar axis'

%% add in external forces and moments here
phidotdot = (M(1) + disc.Id*q*p*sin(theta) - disc.Ia*q*(p*sin(theta)+r) + disc.Id*q*p*sin(theta))/disc.Id/cos(theta); 
thetadotdot = (M(2) + disc.Ia*p*cos(theta)*(p*sin(theta) +r) - disc.Id*p*p*cos(theta)*sin(theta))/disc.Id;
gammadotdot = (M(3) - disc.Ia*(r*sin(theta) + q*p*cos(theta)))/disc.Ia;

% bug in hummels report?
% gammadotdot = (M(3) - disc.Ia*(phidotdot*sin(theta) + thetadot*phidot*cos(theta)))/disc.Ia;
% bug in hummels report?
% w/phidotdot term, there is no decay in gammadot
% w/out gammadot term - there is no decay in gammadot
% NOTE: w/it, the decay is too agressive
% FIXME: investigate why this term is necessary for more appropriate
% spindown (based on my data)

%%
% dTHdt2(1) = p;
% dTHdt2(2) = q;
% dTHdt2(3) = r;

dTHdt2(1) = phidotdot;
dTHdt2(2) = thetadotdot;
dTHdt2(3) = gammadotdot;

== matlab function flatball_6dof/flatball-6dof-HandH/calc-F-M/calc-alpha/calc-alpha ==
  data: dXdt input; alpha output; T_c_N input
function alpha  = f( dXdt, T_c_N)
%% internal states
u = dXdt(1); v = dXdt(2); w = dXdt(3);

%% helper variables
T_c_Npsi = T_c_N(3,:);

vel = [u v w];
vc3 = dot( vel, T_c_Npsi);
v_N = vel - vc3*T_c_Npsi;

alpha = atan( vc3 / norm( v_N)); % angle of attack

== matlab function flatball_6dof/flatball-6dof-HandH/Subsystem/attitude-transform ==
  data: T output; TH input
function T = Ta( TH)
% attitude transformation per Etkin and Reid 1995
phi = TH(1); theta = TH(2); psi = TH(3);
T = [
    cos(theta)*cos(psi), sin(phi)*sin(theta)*cos(psi) - cos(phi)*sin(psi), cos(phi)*sin(theta)*cos(psi) + sin(phi)*sin(psi);
    cos(theta)*sin(psi), sin(phi)*sin(theta)*sin(psi) + cos(phi)*cos(psi), cos(phi)*sin(theta)*sin(psi) - sin(phi)*cos(psi);
    -sin(theta), sin(phi)*cos(theta), cos(phi)*cos(theta)
    ];

== matlab function flatball_6dof/flatball-6dof-HandH/calc-F-M/calc-F/calc-F ==
  data: vel input; F output; T_c_N input; Fg_N input; CLift input; CDrag input; q_inf_times_S input; lift output; drag output; vmag output
function [F, lift, drag, vmag] = fcn( vel, T_c_N, Fg_N, CLift, CDrag, q_inf_times_S)
%%
T_c_Npsi = T_c_N(3,:);

vc3 = dot( vel', T_c_Npsi);
v_N = vel' - vc3*T_c_Npsi;
vmag = norm( vel');
uvel = vel' / vmag;
uv_N = v_N / norm( v_N);
u_lat = cross( T_c_Npsi, uv_N);

lift = CLift * q_inf_times_S;
ulift = -cross( uvel, u_lat);

drag = CDrag * q_inf_times_S;
udrag = -uvel;

Faero = lift*ulift + drag*udrag;

F = Faero' + Fg_N;

== matlab function flatball_6dof/flatball-6dof-HandH/Subsystem/rate-transform ==
  data: T output; TH input
function T = Tr( TH)
% euler angle rate transformation per Etkin and Reid 1995
phi = TH(1); theta = TH(2); % psi = TH(3);
T = [
    1, sin(phi)*tan(theta), cos(phi)*tan(theta);
    0, cos(phi), -sin(phi);
    0, sin(phi)*sec(theta), cos(phi)*sec(theta)
    ];

== matlab function flatball_6dof/flatball-6dof-HandH/calc-F-M/calc-F/q-inf/vector-norm ==
  data: vec input; norm output
function norm = fcn( vec)

norm = sqrt( vec(1)*vec(1) + vec(2)*vec(2) + vec(3)*vec(3));

== matlab function flatball_6dof/flatball-6dof-HandH/calc-Xdot1/calc-THdot ==
  data: X input; M input; dTHdt2 output; Mlaunch input
function dTHdt2   = f_rot( X, M, Mlaunch)
% flatball equations of motion - NED (north-east-down) configuration
%

%% internal states
phi = X(4); theta = X(5); gamma = X(6);
p = X(10); q = X(11); r = X(12);

dTHdt2 = zeros(3,1);

%% define non-aerodynamic parameters
disc = struct;
disc.Ia = 0.002352; % moment of inertia about the spinning axis
disc.Id = 0.001219; % moment of inertia about the planar axis'

%% add in external forces and moments here
phidotdot = ((M(1) + Mlaunch(1)) + disc.Id*q*p*sin(theta) - disc.Ia*q*(p*sin(theta)+r) + disc.Id*q*p*sin(theta))/disc.Id/cos(theta); 
thetadotdot = ((M(2) + Mlaunch(2)) + disc.Ia*p*cos(theta)*(p*sin(theta) +r) - disc.Id*p*p*cos(theta)*sin(theta))/disc.Id;
gammadotdot = ((M(3) + Mlaunch(3)) - disc.Ia*(r*sin(theta) + q*p*cos(theta)))/disc.Ia;

% bug in hummels report?
% gammadotdot = (M(3) - disc.Ia*(phidotdot*sin(theta) + thetadot*phidot*cos(theta)))/disc.Ia;
% bug in hummels report?
% w/phidotdot term, there is no decay in gammadot
% w/out gammadot term - there is no decay in gammadot
% NOTE: w/it, the decay is too agressive
% FIXME: investigate why this term is necessary for more appropriate
% spindown (based on my data)

%%
% dTHdt2(1) = p;
% dTHdt2(2) = q;
% dTHdt2(3) = r;

dTHdt2(1) = phidotdot;
dTHdt2(2) = thetadotdot;
dTHdt2(3) = gammadotdot;
